simulink model "svpwm_realize"  (R2019b)
settings: Solver=FixedStepAuto  StartTime=0.0  StopTime=0.1  FixedStep=To  RelTol=1e-3
values from neighbouring files (symbols this model uses):
  Amp = 1    [m_svpwm_npc.m]
  Ts = 1/Fs    (= 5e-05)    [m_svpwm_npc.m]
libraries: simulink_extras x1, powerlib x1
settings Model: Creator=Dmitry  LastModifiedBy=NPT

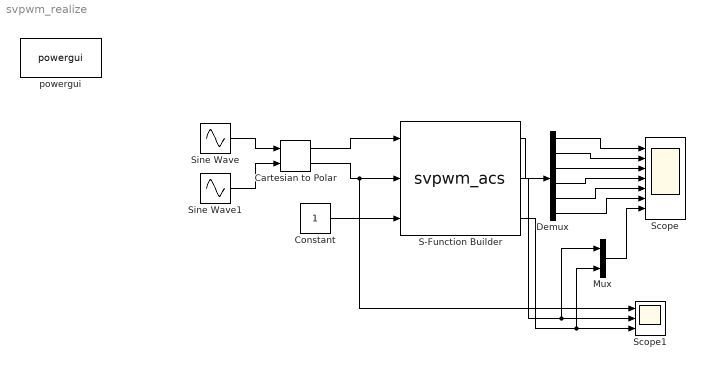
== system svpwm_realize ==
  Cartesian to Polar : simulink_extras/Transformations/Cartesian to Polar
      settings: SourceProductName=Simulink
  Constant : Constant
  Demux : Demux  Outputs=6
  Mux : Mux  Inputs=2
  S-Function Builder : S-Function  InitFcn=try, set_param(gcb,'FunctionName','svpwm_acs'), end  FunctionName=svpwm_acs  Parameters=Ts  SFunctionModules=svpwm_acs_wrapper CSVPWM_NPC  SFunctionDeploymentMode=off  EnableBusSupport=off  mask(S-Function Builder){}
      mask help: Simulink:masks:SFunctionBuilder_MD
      mask init:
      | val = [[.9  0.75 0.75 1 1 .9 .9 1]',[1 1 0.75 0.75 .9 .9 1 .9]'];try , sys = get_param(gcb,'SfunBuilderFcnName');if isempty(sys), sys = get_param(gcb,'FunctionName'); end,catch, sys = get_param(gcb,'FunctionName'); end
      settings: CopyFcn=set_param(gcbh,'LinkStatus','none')  PreSaveFcn=try, set_param(gcb,'FunctionName','svpwm_acs'), end  OpenFcn=sfunctionwizard(gcbh)
      mask Display:
      | plot(val(:,1),val(:,2))
      | disp(sys)
      | port_label('input',1,'mag')
      | port_label('input',2,'th')
      | port_label('input',3,'selCap')
      | port_label('output',1,'ccr')
      | port_label('output',2,'sctr')
      | port_label('output',3,'subsctr')
  Scope : Scope  NumInputPorts=7
  Scope1 : Scope  NumInputPorts=3
  Sine Wave : Sin  Amplitude=Amp  Frequency=100*pi  Phase=pi/2  SampleTime=Ts
  Sine Wave1 : Sin  Amplitude=Amp  Frequency=100*pi  SampleTime=Ts
  powergui : powerlib/powergui  Priority=1  SimulationMode=Discrete  SampleTime=50e-6  frequency=60  Iterations=50  frequencyindice=60  Pbase=100e6  ErrMax=1e-4  UnitsV=kV  UnitsW=MW  buscounter=0  FunctionMessages=off  echomessages=off  EnableUseOfTLC=off  CurrentSourceSwitches=off  DisableSnubberDevices=off  DisableRonSwitches=off  DisableVfSwitches=off  DisplayEquations=off  AutomaticDiscreteSolvers=off  SolverType=Tustin/Backward Euler (TBE)  Interpol=off  ExternalGateDelay=off  methode=off  Ts=100  x0status=blocks  SPID=on  SwTol=0  HookPort=off  NonlinearTolerance=1e-4  nMaxIteration=100  ContinueOnMaxIteration=off  RestoreLinks=warning  ResistiveCurrentMeasurement=off  Frange=[0:2:500]  Ylog=off  Xlog=on  ShowGrid=off  save=off  variable=ZData  structure=0  ZoomFFT=off  StartTime=0.0  cycles=1  DisplayStyle=1  fundamental=60  FreqAxis=off  MaxFrequency=1000  frequencyindicesteady=1  RmsSteady=1  display=off
      settings: SourceProductName=Simscape Electrical
  wires:
  Sine Wave/1 -> Cartesian to Polar/1
  Sine Wave1/1 -> Cartesian to Polar/2
  Cartesian to Polar/1 -> S-Function Builder/1
  Cartesian to Polar/2 -> Scope1/1, S-Function Builder/2
  Constant/1 -> S-Function Builder/3
  S-Function Builder/1 -> Demux/1
  Demux/1 -> Scope/1
  Demux/2 -> Scope/2
  Demux/3 -> Scope/3
  Demux/4 -> Scope/4
  Demux/5 -> Scope/5
  Demux/6 -> Scope/6
  S-Function Builder/2 -> Mux/1, Scope1/2
  S-Function Builder/3 -> Mux/2, Scope1/3
  Mux/1 -> Scope/7
